simulink model "Lcontainer_simNN"  (R2018b)
settings: Solver=FixedStepAuto  StartTime=0.0  StopTime=50  FixedStep=0.1  RelTol=1e-3
libraries: neural x548, simulink x2
(part 3 of 26)

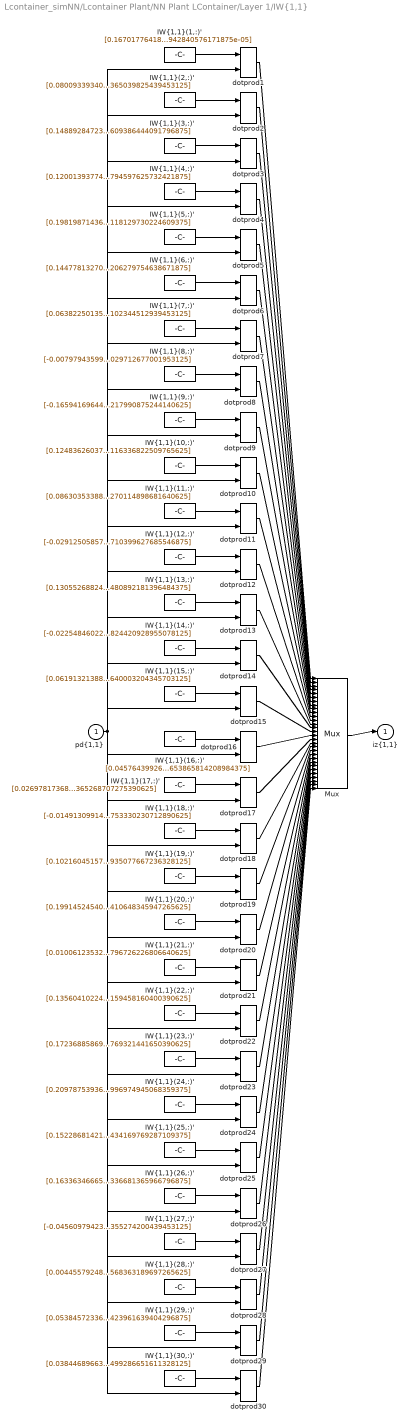
== system Lcontainer_simNN/Lcontainer Plant/NN Plant LContainer/Layer 1/IW{1,1} ==
  "pd{1,1}" : Inport  PortDimensions=10
      mask Display: e = 0.06;c1 = [120 230 180]/255;c2 = ([120 230 180]+0)/(256+128);c3 = ([120 230 180]+128)/(256+128);patch([0 1 1 0],[0 0 1 1],c1);patch([0 1 1 1-e 1-e 0+e],[0 0 1 1-e 0+e 0+e],c2);patch([0 0 1 1-e 0+e 0+e],[0 1 1 1-e 1-e 0+e],c3);plot([0 1 1 0 0],[0 0 1 1 0]);
  "IW{1,1}(1,:)'" : Constant  Value=[0.1670177641811616264799766895521315746009349822998046875;0.01560102160777569225980077050053296261467039585113525390625;0.1353504667630745783579726548850885592401027679443359375;-0.04250494535911998605914874360678368248045444488525390625;0.0684296477871207120546870328325894661247730255126953125;-0.51362198502479172734780377140850760042667388916015625;-0.00801913460694114212101712979574585915543138980865478515625;-0.002839228628072099601398203816415843903087079524993896484375;-0.07313629313567386602823461316802422516047954559326171875;-1.416090249272215271614076825823502758794347755610942840576171875e-05]
      mask Display: e = 0.06;c1 = [120 150 230]/255;c2 = ([120 150 230]+0)/383;c3 = ([120 150 230]+128)/383;patch([0 1 1 0],[0 0 1 1],c1);patch([0 1 1 1-e 1-e 0+e],[0 0 1 1-e 0+e 0+e],c2);patch([0 0 1 1-e 0+e 0+e],[0 1 1 1-e 1-e 0+e],c3);plot([0 1 1 0 0],[0 0 1 1 0]);disp('Weights');
  "IW{1,1}(10,:)'" : Constant  Value=[0.124836260374901752978615832034847699105739593505859375;-0.161949312454792437865336296454188413918018341064453125;-0.1362638506570842122922471162382862530648708343505859375;-0.0926135319083747632351588663368602283298969268798828125;-0.00957801924665558322702363369671729742549359798431396484375;-0.045419427604590577318699473607921390794217586517333984375;0.043044199038925430589319631735634175129234790802001953125;0.139030195333694372994415289213065989315509796142578125;-0.07995932098118506414774486756869009695947170257568359375;0.00092513261988871366148234898219016031362116336822509765625]
      mask Display: e = 0.06;c1 = [120 150 230]/255;c2 = ([120 150 230]+0)/383;c3 = ([120 150 230]+128)/383;patch([0 1 1 0],[0 0 1 1],c1);patch([0 1 1 1-e 1-e 0+e],[0 0 1 1-e 0+e 0+e],c2);patch([0 0 1 1-e 0+e 0+e],[0 1 1 1-e 1-e 0+e],c3);plot([0 1 1 0 0],[0 0 1 1 0]);disp('Weights');
  "IW{1,1}(11,:)'" : Constant  Value=[0.08630353388669521896847669495400623418390750885009765625;-0.1791665087636944153626217257624375633895397186279296875;0.202576576266262409209417683086940087378025054931640625;0.0236792684862243939247772317457929602824151515960693359375;0.0018701201837262593219435302671627141535282135009765625;-0.01483678593335212118897725730448655667714774608612060546875;0.004616789438543386116242661643127576098777353763580322265625;0.17930907263011786056949858902953565120697021484375;-0.08159303040363997949757646210855455137789249420166015625;0.0282039361310799409354732603105730959214270114898681640625]
      mask Display: e = 0.06;c1 = [120 150 230]/255;c2 = ([120 150 230]+0)/383;c3 = ([120 150 230]+128)/383;patch([0 1 1 0],[0 0 1 1],c1);patch([0 1 1 1-e 1-e 0+e],[0 0 1 1-e 0+e 0+e],c2);patch([0 0 1 1-e 0+e 0+e],[0 1 1 1-e 1-e 0+e],c3);plot([0 1 1 0 0],[0 0 1 1 0]);disp('Weights');
  "IW{1,1}(12,:)'" : Constant  Value=[-0.0291250585768351132054387875314205302856862545013427734375;0.00952921702394945481506827178463936434127390384674072265625;0.267259919627413744525057381906663067638874053955078125;-0.0051808169387411208417493213573834509588778018951416015625;0.0174625145621995596367792558112341794185340404510498046875;0.063044600541946216321065321608330123126506805419921875;0.319398294249768899266683774840203113853931427001953125;0.269579842613730746858635711760143749415874481201171875;0.07014645562363795716631642562788329087197780609130859375;0.0264684519642995434718368841231495025567710399627685546875]
      mask Display: e = 0.06;c1 = [120 150 230]/255;c2 = ([120 150 230]+0)/383;c3 = ([120 150 230]+128)/383;patch([0 1 1 0],[0 0 1 1],c1);patch([0 1 1 1-e 1-e 0+e],[0 0 1 1-e 0+e 0+e],c2);patch([0 0 1 1-e 0+e 0+e],[0 1 1 1-e 1-e 0+e],c3);plot([0 1 1 0 0],[0 0 1 1 0]);disp('Weights');
  "IW{1,1}(13,:)'" : Constant  Value=[0.1305526882482727357714935578769654966890811920166015625;-0.06528203150705998158986886892307666130363941192626953125;0.047305218793122140452656054776525706984102725982666015625;0.0136865357230403807131668969532256596721708774566650390625;0.00673344780706026761751825659985115635208785533905029296875;0.03229255147069413911520285864753532223403453826904296875;0.41348167507024446987173860179609619081020355224609375;0.027804499625473745594295138516827137209475040435791015625;-0.2340958545503011023480866015233914367854595184326171875;0.004478330805760355991240739825798300444148480892181396484375]
      mask Display: e = 0.06;c1 = [120 150 230]/255;c2 = ([120 150 230]+0)/383;c3 = ([120 150 230]+128)/383;patch([0 1 1 0],[0 0 1 1],c1);patch([0 1 1 1-e 1-e 0+e],[0 0 1 1-e 0+e 0+e],c2);patch([0 0 1 1-e 0+e 0+e],[0 1 1 1-e 1-e 0+e],c3);plot([0 1 1 0 0],[0 0 1 1 0]);disp('Weights');
  "IW{1,1}(14,:)'" : Constant  Value=[-0.0225484602282647710047580602576999808661639690399169921875;0.05774873566135345359651154240054893307387828826904296875;0.5060283476829223747728292437386699020862579345703125;0.0159029837915102383039123168373407679609954357147216796875;0.02838772171995175563896651738104992546141147613525390625;0.1965938960797436185767850247430033050477504730224609375;0.007917434912395042434507530515475082211196422576904296875;0.1518871622845466007323267376705189235508441925048828125;-0.0247704620376429270056650722153790411539375782012939453125;0.041300061479661316632405743121125851757824420928955078125]
      mask Display: e = 0.06;c1 = [120 150 230]/255;c2 = ([120 150 230]+0)/383;c3 = ([120 150 230]+128)/383;patch([0 1 1 0],[0 0 1 1],c1);patch([0 1 1 1-e 1-e 0+e],[0 0 1 1-e 0+e 0+e],c2);patch([0 0 1 1-e 0+e 0+e],[0 1 1 1-e 1-e 0+e],c3);plot([0 1 1 0 0],[0 0 1 1 0]);disp('Weights');
  "IW{1,1}(15,:)'" : Constant  Value=[0.061913213887811104074732071467224159277975559234619140625;-0.0216362295870577703293946569829131476581096649169921875;0.101317485680977592554796729018562473356723785400390625;0.0210881847815000689205788830804522149264812469482421875;0.00696638032098011172887908060147310607135295867919921875;0.11983017463584390294162318468806915916502475738525390625;0.239337512403481167400087770147365517914295196533203125;-0.1171358792934586168232868885752395726740360260009765625;0.398774716873063372890584332708385773003101348876953125;0.038324897351688147484338742287945933640003204345703125]
      mask Display: e = 0.06;c1 = [120 150 230]/255;c2 = ([120 150 230]+0)/383;c3 = ([120 150 230]+128)/383;patch([0 1 1 0],[0 0 1 1],c1);patch([0 1 1 1-e 1-e 0+e],[0 0 1 1-e 0+e 0+e],c2);patch([0 0 1 1-e 0+e 0+e],[0 1 1 1-e 1-e 0+e],c3);plot([0 1 1 0 0],[0 0 1 1 0]);disp('Weights');
  "IW{1,1}(16,:)'" : Constant  Value=[0.04576439926106130873240118717149016447365283966064453125;0.137842889518047184704840901758871041238307952880859375;-0.001062896226088540056753384277499208110384643077850341796875;0.000427366088309317419639821178378724653157405555248260498046875;0.028343598215901218140277961765605141408741474151611328125;0.0991572984578191485294240692383027635514736175537109375;0.006167476552930396642426824627136738854460418224334716796875;0.1762641333075480598591155967369559220969676971435546875;-0.204617122673511175889871083199977874755859375;0.0200528267813603854052839636779026477597653865814208984375]
      mask Display: e = 0.06;c1 = [120 150 230]/255;c2 = ([120 150 230]+0)/383;c3 = ([120 150 230]+128)/383;patch([0 1 1 0],[0 0 1 1],c1);patch([0 1 1 1-e 1-e 0+e],[0 0 1 1-e 0+e 0+e],c2);patch([0 0 1 1-e 0+e 0+e],[0 1 1 1-e 1-e 0+e],c3);plot([0 1 1 0 0],[0 0 1 1 0]);disp('Weights');
  "IW{1,1}(17,:)'" : Constant  Value=[0.026978173681238150349859239440775127150118350982666015625;-0.2174714602322888323815419653328717686235904693603515625;-0.324306484500667069337254133643000386655330657958984375;0.019968231199915954798829176297658705152571201324462890625;0.0183235476946951754417813873487830278463661670684814453125;0.12304325953026350182195614024749374948441982269287109375;0.07645980262426817219978403272762079723179340362548828125;0.156011582504076873334497577161528170108795166015625;0.3010074819622747810399232548661530017852783203125;-0.000943885662108405313654169166426299852901138365268707275390625]
      mask Display: e = 0.06;c1 = [120 150 230]/255;c2 = ([120 150 230]+0)/383;c3 = ([120 150 230]+128)/383;patch([0 1 1 0],[0 0 1 1],c1);patch([0 1 1 1-e 1-e 0+e],[0 0 1 1-e 0+e 0+e],c2);patch([0 0 1 1-e 0+e 0+e],[0 1 1 1-e 1-e 0+e],c3);plot([0 1 1 0 0],[0 0 1 1 0]);disp('Weights');
  "IW{1,1}(18,:)'" : Constant  Value=[-0.01491309914457791645225892551707147504203021526336669921875;0.004544201607269822418277982478684862144291400909423828125;-0.01445748639927858965326112894445031997747719287872314453125;-0.00997202094028175160811411359418343636207282543182373046875;-0.056222949623621787385019388239015825092792510986328125;-0.10192838113112891174072416333729051984846591949462890625;-0.015872460559222194287354312791649135760962963104248046875;0.0052542880674311086275363180675412877462804317474365234375;-0.0033113225924444136295810015013785232440568506717681884765625;-0.007569031934165791099256015428409227752126753330230712890625]
      mask Display: e = 0.06;c1 = [120 150 230]/255;c2 = ([120 150 230]+0)/383;c3 = ([120 150 230]+128)/383;patch([0 1 1 0],[0 0 1 1],c1);patch([0 1 1 1-e 1-e 0+e],[0 0 1 1-e 0+e 0+e],c2);patch([0 0 1 1-e 0+e 0+e],[0 1 1 1-e 1-e 0+e],c3);plot([0 1 1 0 0],[0 0 1 1 0]);disp('Weights');
  "IW{1,1}(19,:)'" : Constant  Value=[0.102160451576448263466545540723018348217010498046875;0.1056481880648582893922338143966044299304485321044921875;-0.1366538710795570654710218150285072624683380126953125;0.0016875852705349812625523764353374644997529685497283935546875;0.0266990065681217449145012921007946715690195560455322265625;-0.1707127678418920713188100535262492485344409942626953125;0.1685697706561184727735991373265278525650501251220703125;0.00947885967350793612329340476208017207682132720947265625;-0.0174334840764413141755984071323837270028889179229736328125;-0.008740802388134523426277411317641963250935077667236328125]
      mask Display: e = 0.06;c1 = [120 150 230]/255;c2 = ([120 150 230]+0)/383;c3 = ([120 150 230]+128)/383;patch([0 1 1 0],[0 0 1 1],c1);patch([0 1 1 1-e 1-e 0+e],[0 0 1 1-e 0+e 0+e],c2);patch([0 0 1 1-e 0+e 0+e],[0 1 1 1-e 1-e 0+e],c3);plot([0 1 1 0 0],[0 0 1 1 0]);disp('Weights');
  "IW{1,1}(2,:)'" : Constant  Value=[0.08009339340274156116006309957811026833951473236083984375;-0.341187651594337726379535524756647646427154541015625;0.37131085830534249492274057047325186431407928466796875;0.0276570396628715679809840111147423158399760723114013671875;-0.0176590584667420287534600475964907673187553882598876953125;-0.20793086683045325369079137090011499822139739990234375;-0.147240611428952672401493373399716801941394805908203125;0.501763948574379892164643024443648755550384521484375;0.1585647023167238156560188144794665277004241943359375;-0.0050605043202657691570056641694463905878365039825439453125]
      mask Display: e = 0.06;c1 = [120 150 230]/255;c2 = ([120 150 230]+0)/383;c3 = ([120 150 230]+128)/383;patch([0 1 1 0],[0 0 1 1],c1);patch([0 1 1 1-e 1-e 0+e],[0 0 1 1-e 0+e 0+e],c2);patch([0 0 1 1-e 0+e 0+e],[0 1 1 1-e 1-e 0+e],c3);plot([0 1 1 0 0],[0 0 1 1 0]);disp('Weights');
  "IW{1,1}(20,:)'" : Constant  Value=[0.1991452454039419894815665657006320543587207794189453125;-0.1956424860890517980482883331205812282860279083251953125;-0.00701963429226160236240605883040188928134739398956298828125;-0.0112617468728325280380442308114652405492961406707763671875;-0.0267009858683903457399200220834245556034147739410400390625;-0.336474863993861728062029214925132691860198974609375;0.137435633543130764078199490541010163724422454833984375;0.148090412697930273733248895950964652001857757568359375;-0.1631223921012745770031671099786763079464435577392578125;-0.004046200557424725098576434589858763501979410648345947265625]
      mask Display: e = 0.06;c1 = [120 150 230]/255;c2 = ([120 150 230]+0)/383;c3 = ([120 150 230]+128)/383;patch([0 1 1 0],[0 0 1 1],c1);patch([0 1 1 1-e 1-e 0+e],[0 0 1 1-e 0+e 0+e],c2);patch([0 0 1 1-e 0+e 0+e],[0 1 1 1-e 1-e 0+e],c3);plot([0 1 1 0 0],[0 0 1 1 0]);disp('Weights');
  "IW{1,1}(21,:)'" : Constant  Value=[0.0100612353260697666434975161564580048434436321258544921875;-0.047758173787906567364647258955301367677748203277587890625;0.08753622655184885303913944198939134366810321807861328125;-0.01203498314183600211013658309866514173336327075958251953125;0.039696154668679768662276075019690324552357196807861328125;0.061552473494788033370195279303516144864261150360107421875;-0.159032940766079933236909482729970477521419525146484375;0.22249948469810387763345715939067304134368896484375;-0.053958295229308998741668546017535845749080181121826171875;0.0261808854632667765971465456686928519047796726226806640625]
      mask Display: e = 0.06;c1 = [120 150 230]/255;c2 = ([120 150 230]+0)/383;c3 = ([120 150 230]+128)/383;patch([0 1 1 0],[0 0 1 1],c1);patch([0 1 1 1-e 1-e 0+e],[0 0 1 1-e 0+e 0+e],c2);patch([0 0 1 1-e 0+e 0+e],[0 1 1 1-e 1-e 0+e],c3);plot([0 1 1 0 0],[0 0 1 1 0]);disp('Weights');
  "IW{1,1}(22,:)'" : Constant  Value=[0.1356041022414495866854622363462112843990325927734375;0.0287949137235390360822773203608448966406285762786865234375;-0.05502970772566261048464042460182099603116512298583984375;0.0241051437300884539849388232823912403546273708343505859375;0.0311590884976121473837196163003682158887386322021484375;-0.3048121330609430135183401944232173264026641845703125;-0.042395171411425285057372747132831136696040630340576171875;0.33841889538137248649718458182178437709808349609375;0.08028790925315244797477731708568171598017215728759765625;0.01016868751942316163872082057650914066471159458160400390625]
      mask Display: e = 0.06;c1 = [120 150 230]/255;c2 = ([120 150 230]+0)/383;c3 = ([120 150 230]+128)/383;patch([0 1 1 0],[0 0 1 1],c1);patch([0 1 1 1-e 1-e 0+e],[0 0 1 1-e 0+e 0+e],c2);patch([0 0 1 1-e 0+e 0+e],[0 1 1 1-e 1-e 0+e],c3);plot([0 1 1 0 0],[0 0 1 1 0]);disp('Weights');
  "IW{1,1}(23,:)'" : Constant  Value=[0.17236885869881424238059253184474073350429534912109375;0.047838557391975740362699553998027113266289234161376953125;0.292485349552997764277506576036103069782257080078125;-0.01494905367260888039149246964143458171747624874114990234375;0.0022834452479763641015442221515741039183922111988067626953125;-0.410351306603296495101318441811599768698215484619140625;0.31149635452079904585076519651920534670352935791015625;-0.387317499844863244451431683046394027769565582275390625;0.1658780973017434379190859772279509343206882476806640625;0.0204665685198074688566638457132285111583769321441650390625]
      mask Display: e = 0.06;c1 = [120 150 230]/255;c2 = ([120 150 230]+0)/383;c3 = ([120 150 230]+128)/383;patch([0 1 1 0],[0 0 1 1],c1);patch([0 1 1 1-e 1-e 0+e],[0 0 1 1-e 0+e 0+e],c2);patch([0 0 1 1-e 0+e 0+e],[0 1 1 1-e 1-e 0+e],c3);plot([0 1 1 0 0],[0 0 1 1 0]);disp('Weights');
  "IW{1,1}(24,:)'" : Constant  Value=[0.2097875393615591665952280209239688701927661895751953125;-0.09495759574741362285532630949091981165111064910888671875;-0.1285436793632044605306674611711059696972370147705078125;0.01222204376306920865780103468978268210776150226593017578125;0.044848969988143756737475342788457055576145648956298828125;0.171455733638167184818001942403498105704784393310546875;0.1716821094202888031698961412985227070748805999755859375;-0.254982212662857310458974779976415447890758514404296875;-0.173045137444410912497261278986115939915180206298828125;0.0235080406647079319382154238837756565771996974945068359375]
      mask Display: e = 0.06;c1 = [120 150 230]/255;c2 = ([120 150 230]+0)/383;c3 = ([120 150 230]+128)/383;patch([0 1 1 0],[0 0 1 1],c1);patch([0 1 1 1-e 1-e 0+e],[0 0 1 1-e 0+e 0+e],c2);patch([0 0 1 1-e 0+e 0+e],[0 1 1 1-e 1-e 0+e],c3);plot([0 1 1 0 0],[0 0 1 1 0]);disp('Weights');
  "IW{1,1}(25,:)'" : Constant  Value=[0.1522868142176449224312051455854088999330997467041015625;0.0613446776501501422895756832076585851609706878662109375;-0.310982062171623219182237107816035859286785125732421875;-0.0032237638202379311110068460521915767458267509937286376953125;0.0140840055050879368880867303914783406071364879608154296875;-0.1884296977286029906029085623231367208063602447509765625;0.2030475312449748492849010972349788062274456024169921875;0.05213390281310419094307206933081033639609813690185546875;0.0997416659013728168492463055372354574501514434814453125;0.034861902284974675969575486078610992990434169769287109375]
      mask Display: e = 0.06;c1 = [120 150 230]/255;c2 = ([120 150 230]+0)/383;c3 = ([120 150 230]+128)/383;patch([0 1 1 0],[0 0 1 1],c1);patch([0 1 1 1-e 1-e 0+e],[0 0 1 1-e 0+e 0+e],c2);patch([0 0 1 1-e 0+e 0+e],[0 1 1 1-e 1-e 0+e],c3);plot([0 1 1 0 0],[0 0 1 1 0]);disp('Weights');
  "IW{1,1}(26,:)'" : Constant  Value=[0.1633634666572907623294241830080864019691944122314453125;0.0611842341447732807058201842664857394993305206298828125;-0.0164054417311453142047650288759541581384837627410888671875;0.0303971170781771500568613220139013719744980335235595703125;0.043976399273147094570735049501308822073042392730712890625;0.03222329894874524647274682820352609269320964813232421875;-0.114874120697126935741749775843345560133457183837890625;0.2104153205438100970869896855219849385321140289306640625;-0.32409609917607451468057888632756657898426055908203125;0.0276911525214954649942722397781835752539336681365966796875]
      mask Display: e = 0.06;c1 = [120 150 230]/255;c2 = ([120 150 230]+0)/383;c3 = ([120 150 230]+128)/383;patch([0 1 1 0],[0 0 1 1],c1);patch([0 1 1 1-e 1-e 0+e],[0 0 1 1-e 0+e 0+e],c2);patch([0 0 1 1-e 0+e 0+e],[0 1 1 1-e 1-e 0+e],c3);plot([0 1 1 0 0],[0 0 1 1 0]);disp('Weights');
  "IW{1,1}(27,:)'" : Constant  Value=[-0.0456097942352748919603300237213261425495147705078125;-0.038990227588823721249777776165501563809812068939208984375;0.1190274353800651052637249449617229402065277099609375;0.044440348726322624617335321772770839743316173553466796875;-0.0157334614524682163405611134976425091736018657684326171875;0.2528380731518364843424251375836320221424102783203125;0.1443586450668634946215007630598847754299640655517578125;0.169663623456062950811684686414082534611225128173828125;-0.060544000159965916108006922513595782220363616943359375;-0.006532667738801779984403328427333690342493355274200439453125]
      mask Display: e = 0.06;c1 = [120 150 230]/255;c2 = ([120 150 230]+0)/383;c3 = ([120 150 230]+128)/383;patch([0 1 1 0],[0 0 1 1],c1);patch([0 1 1 1-e 1-e 0+e],[0 0 1 1-e 0+e 0+e],c2);patch([0 0 1 1-e 0+e 0+e],[0 1 1 1-e 1-e 0+e],c3);plot([0 1 1 0 0],[0 0 1 1 0]);disp('Weights');
  "IW{1,1}(28,:)'" : Constant  Value=[0.004455792481407373252511039396495107212103903293609619140625;-0.1525799045239943085849887438598670996725559234619140625;-0.181958083684146398883996198492241092026233673095703125;0.008669723737217048531444874015505774877965450286865234375;0.01396507172824217567208560097924419096671044826507568359375;0.282196644384983541531397577273310162127017974853515625;0.1723855130708553395901816429613973014056682586669921875;0.03867984891526025925667653382333810441195964813232421875;0.116163982107230723261892535447259433567523956298828125;0.016602825390363208646338222251870320178568363189697265625]
      mask Display: e = 0.06;c1 = [120 150 230]/255;c2 = ([120 150 230]+0)/383;c3 = ([120 150 230]+128)/383;patch([0 1 1 0],[0 0 1 1],c1);patch([0 1 1 1-e 1-e 0+e],[0 0 1 1-e 0+e 0+e],c2);patch([0 0 1 1-e 0+e 0+e],[0 1 1 1-e 1-e 0+e],c3);plot([0 1 1 0 0],[0 0 1 1 0]);disp('Weights');
  "IW{1,1}(29,:)'" : Constant  Value=[0.053845723365219290423855369454031460918486118316650390625;0.32789251100956973150601925226510502398014068603515625;-0.03728070715760194164811736072806525044143199920654296875;0.040818200014749554671578124498410033993422985076904296875;0.00077892276380062304419471530536611680872738361358642578125;0.0748344604920810618775561806614859960973262786865234375;0.08365982952625160284920724507173872552812099456787109375;0.0735423990272566496795292323440662585198879241943359375;0.05504566822072075316096828601075685583055019378662109375;0.046737770425980595945247841882519423961639404296875]
      mask Display: e = 0.06;c1 = [120 150 230]/255;c2 = ([120 150 230]+0)/383;c3 = ([120 150 230]+128)/383;patch([0 1 1 0],[0 0 1 1],c1);patch([0 1 1 1-e 1-e 0+e],[0 0 1 1-e 0+e 0+e],c2);patch([0 0 1 1-e 0+e 0+e],[0 1 1 1-e 1-e 0+e],c3);plot([0 1 1 0 0],[0 0 1 1 0]);disp('Weights');
  "IW{1,1}(3,:)'" : Constant  Value=[0.1488928472368342970089116761300829239189624786376953125;-0.10820117407079789251245216519237146712839603424072265625;0.02389074054508168176713667207877733744680881500244140625;0.03901871660008582320955383693217299878597259521484375;0.00861987964663078580496158309642851236276328563690185546875;0.1613605083051272703897893734392710030078887939453125;0.205816652571092550960685230165836401283740997314453125;-0.1271492178061756905815826712569105438888072967529296875;-0.22135453122176496076889407049748115241527557373046875;0.006623778514760337958466873686802500742487609386444091796875]
      mask Display: e = 0.06;c1 = [120 150 230]/255;c2 = ([120 150 230]+0)/383;c3 = ([120 150 230]+128)/383;patch([0 1 1 0],[0 0 1 1],c1);patch([0 1 1 1-e 1-e 0+e],[0 0 1 1-e 0+e 0+e],c2);patch([0 0 1 1-e 0+e 0+e],[0 1 1 1-e 1-e 0+e],c3);plot([0 1 1 0 0],[0 0 1 1 0]);disp('Weights');
  "IW{1,1}(30,:)'" : Constant  Value=[0.038446896631665748722550546290221973322331905364990234375;-0.043543063534170860229277622011068160645663738250732421875;0.056669798097712720252872031778679229319095611572265625;0.029897953454220409230668309419343131594359874725341796875;0.0474019869848068264861495890727383084595203399658203125;-0.51761076731059618705188540843664668500423431396484375;-0.0002850323176249772681722927103464826359413564205169677734375;-0.0025172087598511506956189265338252880610525608062744140625;-0.00991883374777240665876032466030665091238915920257568359375;-0.0002108316994517340820132489387361829358269460499286651611328125]
      mask Display: e = 0.06;c1 = [120 150 230]/255;c2 = ([120 150 230]+0)/383;c3 = ([120 150 230]+128)/383;patch([0 1 1 0],[0 0 1 1],c1);patch([0 1 1 1-e 1-e 0+e],[0 0 1 1-e 0+e 0+e],c2);patch([0 0 1 1-e 0+e 0+e],[0 1 1 1-e 1-e 0+e],c3);plot([0 1 1 0 0],[0 0 1 1 0]);disp('Weights');
  "IW{1,1}(4,:)'" : Constant  Value=[0.12001393774693082383553388581276522018015384674072265625;0.004548220639106741007562373368955377372913062572479248046875;-0.033953216913745899729892840923639596439898014068603515625;0.010792687895584129886827895461465232074260711669921875;0.044655713631387240758474632684738026000559329986572265625;0.0448789394996856605413171337204403243958950042724609375;-0.152289752253815968696670779536361806094646453857421875;-0.1753580918527764820336045659132651053369045257568359375;0.27226191519129072649008094231248833239078521728515625;0.047057587951252193014806124438109691254794597625732421875]
      mask Display: e = 0.06;c1 = [120 150 230]/255;c2 = ([120 150 230]+0)/383;c3 = ([120 150 230]+128)/383;patch([0 1 1 0],[0 0 1 1],c1);patch([0 1 1 1-e 1-e 0+e],[0 0 1 1-e 0+e 0+e],c2);patch([0 0 1 1-e 0+e 0+e],[0 1 1 1-e 1-e 0+e],c3);plot([0 1 1 0 0],[0 0 1 1 0]);disp('Weights');
  "IW{1,1}(5,:)'" : Constant  Value=[0.19819871436389335794814314795075915753841400146484375;-0.04874750469319395762557434181871940381824970245361328125;-0.032978259164360167188245753777664504013955593109130859375;0.09739303653778917657657387962899520061910152435302734375;-0.0468123142042608797463998371313209645450115203857421875;-0.314613298456907275468807938523241318762302398681640625;-0.062375528109896584416649290005807415582239627838134765625;-0.00706436138290223412938839686603387235663831233978271484375;-0.044802349287920852083377809549347148276865482330322265625;0.04667125777006386755374478525482118129730224609375]
      mask Display: e = 0.06;c1 = [120 150 230]/255;c2 = ([120 150 230]+0)/383;c3 = ([120 150 230]+128)/383;patch([0 1 1 0],[0 0 1 1],c1);patch([0 1 1 1-e 1-e 0+e],[0 0 1 1-e 0+e 0+e],c2);patch([0 0 1 1-e 0+e 0+e],[0 1 1 1-e 1-e 0+e],c3);plot([0 1 1 0 0],[0 0 1 1 0]);disp('Weights');
  "IW{1,1}(6,:)'" : Constant  Value=[0.144778132701500583667808541576960124075412750244140625;-0.272083384406595463200773110656882636249065399169921875;-0.2468607327036266563258237738409661687910556793212890625;0.016899680997736123144736808399102301336824893951416015625;-0.006347449146304002566554292030787109979428350925445556640625;-0.12089184689880456968769095738025498576462268829345703125;0.26339901999467285609313194072456099092960357666015625;-0.0038042601448462572306941087418863389757461845874786376953125;0.06546144845865183026223377282803994603455066680908203125;0.0187507456483207816944069890041646431200206279754638671875]
      mask Display: e = 0.06;c1 = [120 150 230]/255;c2 = ([120 150 230]+0)/383;c3 = ([120 150 230]+128)/383;patch([0 1 1 0],[0 0 1 1],c1);patch([0 1 1 1-e 1-e 0+e],[0 0 1 1-e 0+e 0+e],c2);patch([0 0 1 1-e 0+e 0+e],[0 1 1 1-e 1-e 0+e],c3);plot([0 1 1 0 0],[0 0 1 1 0]);disp('Weights');
  "IW{1,1}(7,:)'" : Constant  Value=[0.0638225013553249398423616867148666642606258392333984375;-0.034003757460756393882217452073746244423091411590576171875;0.05259656731297450427131678907244349829852581024169921875;0.011875101898354438467730886941353674046695232391357421875;0.05876447230764940410363550427064183168113231658935546875;-0.39444160782916404262010701131657697260379791259765625;0.00527418082020121754827091109518732992000877857208251953125;-0.0089050196112641887002947527207652456127107143402099609375;-0.05825975622805841525053693885638494975864887237548828125;-0.0004195139412729522072897925255574591574259102344512939453125]
      mask Display: e = 0.06;c1 = [120 150 230]/255;c2 = ([120 150 230]+0)/383;c3 = ([120 150 230]+128)/383;patch([0 1 1 0],[0 0 1 1],c1);patch([0 1 1 1-e 1-e 0+e],[0 0 1 1-e 0+e 0+e],c2);patch([0 0 1 1-e 0+e 0+e],[0 1 1 1-e 1-e 0+e],c3);plot([0 1 1 0 0],[0 0 1 1 0]);disp('Weights');
  "IW{1,1}(8,:)'" : Constant  Value=[-0.00797943599061243756531691673217210336588323116302490234375;-0.037971561811335874381256871856749057769775390625;0.0287222418567455277382816092313078115694224834442138671875;-0.07862656964184122632133266961318440735340118408203125;0.002412182210996739739616856468273908831179141998291015625;-0.022119223166929657953261312286485917866230010986328125;-0.00151783068382511346534891050197302320157177746295928955078125;-0.040190306144319544456866566406461060978472232818603515625;0.000949851736959107600076490651730409808806143701076507568359375;-0.00924341817169467734605081687959682312794029712677001953125]
      mask Display: e = 0.06;c1 = [120 150 230]/255;c2 = ([120 150 230]+0)/383;c3 = ([120 150 230]+128)/383;patch([0 1 1 0],[0 0 1 1],c1);patch([0 1 1 1-e 1-e 0+e],[0 0 1 1-e 0+e 0+e],c2);patch([0 0 1 1-e 0+e 0+e],[0 1 1 1-e 1-e 0+e],c3);plot([0 1 1 0 0],[0 0 1 1 0]);disp('Weights');
  "IW{1,1}(9,:)'" : Constant  Value=[-0.16594169644528322660192998228012584149837493896484375;0.1697357264392223286098015933021088130772113800048828125;0.0889545508085859137903383953016600571572780609130859375;0.00176539944569670411399220366632789591676555573940277099609375;-0.0269583024513031337121571340276204864494502544403076171875;0.52799789127653762310643514865660108625888824462890625;0.0176388053434961035448313992901603342033922672271728515625;0.001453740352484169696956062267645393148995935916900634765625;-0.07256776646312430856244901633544941432774066925048828125;0.0004277781714893307885884399244247333626844920217990875244140625]
      mask Display: e = 0.06;c1 = [120 150 230]/255;c2 = ([120 150 230]+0)/383;c3 = ([120 150 230]+128)/383;patch([0 1 1 0],[0 0 1 1],c1);patch([0 1 1 1-e 1-e 0+e],[0 0 1 1-e 0+e 0+e],c2);patch([0 0 1 1-e 0+e 0+e],[0 1 1 1-e 1-e 0+e],c3);plot([0 1 1 0 0],[0 0 1 1 0]);disp('Weights');
  Mux : Mux  Inputs=30
      mask Display: e = 0.06;c1 = [120 150 230]/255;c2 = ([120 150 230]+0)/383;c3 = ([120 150 230]+128)/383;patch([0 1 1 0],[0 0 1 1],c1);patch([0 1 1 1-e 1-e 0+e],[0 0 1 1-e 0+e 0+e],c2);patch([0 0 1 1-e 0+e 0+e],[0 1 1 1-e 1-e 0+e],c3);plot([0 1 1 0 0],[0 0 1 1 0]);disp('Mux');
  dotprod{1..30} (30 alike) : neural/Weight Functions/dotprod
  "iz{1,1}" : Outport
      mask Display: e = 0.06;c1 = [120 230 180]/255;c2 = ([120 230 180]+0)/(256+128);c3 = ([120 230 180]+128)/(256+128);patch([0 1 1 0],[0 0 1 1],c1);patch([0 1 1 1-e 1-e 0+e],[0 0 1 1-e 0+e 0+e],c2);patch([0 0 1 1-e 0+e 0+e],[0 1 1 1-e 1-e 0+e],c3);plot([0 1 1 0 0],[0 0 1 1 0]);
  wires:
  Mux/1 -> "iz{1,1}"/1
  dotprod30/1 -> Mux/30
  "IW{1,1}(30,:)'"/1 -> dotprod30/1
  dotprod29/1 -> Mux/29
  "IW{1,1}(29,:)'"/1 -> dotprod29/1
  dotprod28/1 -> Mux/28
  "IW{1,1}(28,:)'"/1 -> dotprod28/1
  dotprod27/1 -> Mux/27
  "IW{1,1}(27,:)'"/1 -> dotprod27/1
  dotprod26/1 -> Mux/26
  "IW{1,1}(26,:)'"/1 -> dotprod26/1
  dotprod25/1 -> Mux/25
  "IW{1,1}(25,:)'"/1 -> dotprod25/1
  dotprod24/1 -> Mux/24
  "IW{1,1}(24,:)'"/1 -> dotprod24/1
  dotprod23/1 -> Mux/23
  "IW{1,1}(23,:)'"/1 -> dotprod23/1
  dotprod22/1 -> Mux/22
  "IW{1,1}(22,:)'"/1 -> dotprod22/1
  dotprod21/1 -> Mux/21
  "IW{1,1}(21,:)'"/1 -> dotprod21/1
  dotprod20/1 -> Mux/20
  "IW{1,1}(20,:)'"/1 -> dotprod20/1
  dotprod19/1 -> Mux/19
  "IW{1,1}(19,:)'"/1 -> dotprod19/1
  dotprod18/1 -> Mux/18
  "IW{1,1}(18,:)'"/1 -> dotprod18/1
  dotprod17/1 -> Mux/17
  "IW{1,1}(17,:)'"/1 -> dotprod17/1
  dotprod16/1 -> Mux/16
  "IW{1,1}(16,:)'"/1 -> dotprod16/1
  dotprod15/1 -> Mux/15
  "IW{1,1}(15,:)'"/1 -> dotprod15/1
  dotprod14/1 -> Mux/14
  "IW{1,1}(14,:)'"/1 -> dotprod14/1
  dotprod13/1 -> Mux/13
  "IW{1,1}(13,:)'"/1 -> dotprod13/1
  dotprod12/1 -> Mux/12
  "IW{1,1}(12,:)'"/1 -> dotprod12/1
  dotprod11/1 -> Mux/11
  "IW{1,1}(11,:)'"/1 -> dotprod11/1
  dotprod10/1 -> Mux/10
  "IW{1,1}(10,:)'"/1 -> dotprod10/1
  dotprod9/1 -> Mux/9
  "IW{1,1}(9,:)'"/1 -> dotprod9/1
  dotprod8/1 -> Mux/8
  "IW{1,1}(8,:)'"/1 -> dotprod8/1
  dotprod7/1 -> Mux/7
  "IW{1,1}(7,:)'"/1 -> dotprod7/1
  dotprod6/1 -> Mux/6
  "IW{1,1}(6,:)'"/1 -> dotprod6/1
  dotprod5/1 -> Mux/5
  "IW{1,1}(5,:)'"/1 -> dotprod5/1
  dotprod4/1 -> Mux/4
  "IW{1,1}(4,:)'"/1 -> dotprod4/1
  dotprod3/1 -> Mux/3
  "IW{1,1}(3,:)'"/1 -> dotprod3/1
  dotprod2/1 -> Mux/2
  "IW{1,1}(2,:)'"/1 -> dotprod2/1
  dotprod1/1 -> Mux/1
  "pd{1,1}"/1 -> dotprod30/2, dotprod29/2, dotprod28/2, dotprod27/2, dotprod26/2, dotprod25/2, dotprod24/2, dotprod23/2, dotprod22/2, dotprod21/2, dotprod20/2, dotprod19/2, dotprod18/2, dotprod17/2, dotprod16/2, dotprod15/2, dotprod14/2, dotprod13/2, dotprod12/2, dotprod11/2, dotprod10/2, dotprod9/2, dotprod8/2, dotprod7/2, dotprod6/2, dotprod5/2, dotprod4/2, dotprod3/2, dotprod2/2, dotprod1/2
  "IW{1,1}(1,:)'"/1 -> dotprod1/1

== system Lcontainer_simNN/Lcontainer Plant/NN Plant LContainer/Layer 2/Delays 1 ==
  "p{2}" : Inport  PortDimensions=30
      mask Display: e = 0.06;c1 = [120 230 180]/255;c2 = ([120 230 180]+0)/(256+128);c3 = ([120 230 180]+128)/(256+128);patch([0 1 1 0],[0 0 1 1],c1);patch([0 1 1 1-e 1-e 0+e],[0 0 1 1-e 0+e 0+e],c2);patch([0 0 1 1-e 0+e 0+e],[0 1 1 1-e 1-e 0+e],c3);plot([0 1 1 0 0],[0 0 1 1 0]);
  mux : Mux  Inputs=1
      mask Display: e = 0.06;c1 = [120 150 230]/255;c2 = ([120 150 230]+0)/383;c3 = ([120 150 230]+128)/383;patch([0 1 1 0],[0 0 1 1],c1);patch([0 1 1 1-e 1-e 0+e],[0 0 1 1-e 0+e 0+e],c2);patch([0 0 1 1-e 0+e 0+e],[0 1 1 1-e 1-e 0+e],c3);plot([0 1 1 0 0],[0 0 1 1 0]);disp('Mux')
  "pd{2,1}" : Outport
      mask Display: e = 0.06;c1 = [120 230 180]/255;c2 = ([120 230 180]+0)/(256+128);c3 = ([120 230 180]+128)/(256+128);patch([0 1 1 0],[0 0 1 1],c1);patch([0 1 1 1-e 1-e 0+e],[0 0 1 1-e 0+e 0+e],c2);patch([0 0 1 1-e 0+e 0+e],[0 1 1 1-e 1-e 0+e],c3);plot([0 1 1 0 0],[0 0 1 1 0]);
  wires:
  mux/1 -> "pd{2,1}"/1
  "p{2}"/1 -> mux/1
